simulink model "eurlerAngles_sensor_fusion"  (R2021a)
settings: Solver=FixedStepAuto  StartTime=0.0  StopTime=2000  RelTol=1e-3  EnableMultiTasking=on
undefined symbols (not defined in the file): DiscIntNeverNeededParam
libraries: bbblueCommlib x15, bbblueBasicLib x1, bbblueSensorLib x1
settings Model: ExtModeTrigDuration=100  Creator=Zein  LastModifiedBy=zein
settings SolverCC: AlgebraicLoopSolver=TrustRegion  PositivePriorityOrder=on
settings OptimizationCC: EnhancedBackFolding=on  PassReuseOutputArgsAs=Individual arguments  ZeroExternalMemoryAtStartup=off  ZeroInternalMemoryAtStartup=off  MaxStackSize=64  OptimizeBlockOrder=speed  DifferentSizesBufferReuse=on  OptimizationCustomize=off  EfficientTunableParamExpr=on
settings DebuggingCC: ParameterTunabilityLossMsg=error  SFMachineParentedDataDiag=warning
settings HardwareCC: ProdBitPerPointer=32  ProdBitPerSizeT=32  ProdBitPerPtrDiffT=32  ProdLargestAtomicInteger=Long  ProdLargestAtomicFloat=Double  ProdWordSize=32  ProdHWDeviceType=ARM Compatible->ARM Cortex
settings SFSimCC: MATLABDynamicMemAlloc=off
settings RTWCC: SystemTargetFile=ert.tlc  HardwareBoard=BeagleBone Blue  TLCOptions="-aInlineSetEventsForThisBaseRateFcn=TLC_FALSE -aSuppressMultiTaskScheduler=TLC_FALSE  -aRateBasedStepFcn=0"  TemplateMakefile=ert_default_tmf  Toolchain=GNU GCC BeagleBone Blue
settings CodeAppCC: ForceParamTrailComments=on  IgnoreCustomStorageClasses=off  OperatorAnnotations=on  SimulinkDataObjDesc=on  SFDataObjDesc=on  InsertBlockDesc=on
settings ERTTargetCC: MatFileLogging=on  SupportVariableSizeSignals=on

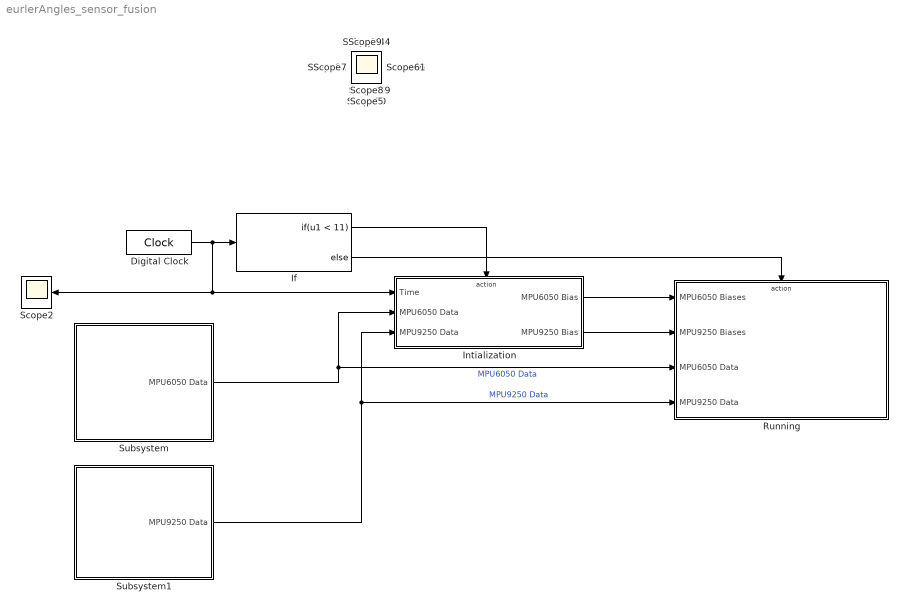
== system eurlerAngles_sensor_fusion ==
  Digital Clock : DigitalClock  SampleTime=0.1
  If : If  IfExpression=u1 < 11
  Intialization : Subsystem  TreatAsAtomicUnit=on
  Running : Subsystem  TreatAsAtomicUnit=on
  Scope{,1..22} (23 alike) : Scope
  Subsystem : Subsystem
  Subsystem1 : Subsystem
  wires:
  If/1 -> Intialization/Action
  Digital Clock/1 -> Scope2/1, Intialization/1(Time), If/1
  If/2 -> Running/Action
  Intialization/1(MPU6050 Bias) -> Running/1(MPU6050 Biases)
  Intialization/2(MPU9250 Bias) -> Running/2(MPU9250 Biases)
  Subsystem/1(MPU6050 Data) -> Intialization/2(MPU6050 Data), Running/3(MPU6050 Data)  "MPU6050 Data"
  Subsystem1/1(MPU9250 Data) -> Intialization/3(MPU9250 Data), Running/4(MPU9250 Data)  "MPU9250 Data"

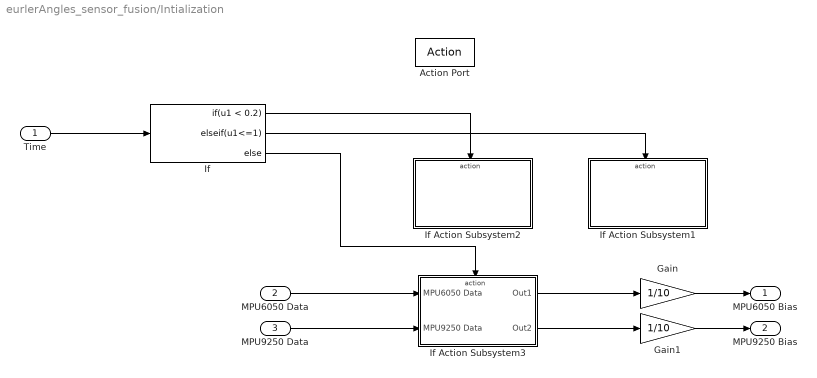
== system eurlerAngles_sensor_fusion/Intialization ==
  Time : Inport
  MPU6050 Data : Inport  Port=2
  MPU9250 Data : Inport  Port=3
  Action Port : ActionPort  ActionPortLabel=if(u1 < 11)
  Gain : Gain  Gain=1/10
  Gain1 : Gain  Gain=1/10
  If : If  IfExpression=u1 < 0.2  ElseIfExpressions=u1<=1
  If Action Subsystem1 : Subsystem  TreatAsAtomicUnit=on
  If Action Subsystem2 : Subsystem  TreatAsAtomicUnit=on
  If Action Subsystem3 : Subsystem  TreatAsAtomicUnit=on
  MPU6050 Bias : Outport
  MPU9250 Bias : Outport  Port=2
  wires:
  Time/1 -> If/1
  If/1 -> If Action Subsystem2/Action
  If/2 -> If Action Subsystem1/Action
  If/3 -> If Action Subsystem3/Action
  If Action Subsystem3/1(Out1) -> Gain/1
  Gain/1 -> MPU6050 Bias/1
  If Action Subsystem3/2(Out2) -> Gain1/1
  Gain1/1 -> MPU9250 Bias/1
  MPU9250 Data/1 -> If Action Subsystem3/2(MPU9250 Data)
  MPU6050 Data/1 -> If Action Subsystem3/1(MPU6050 Data)

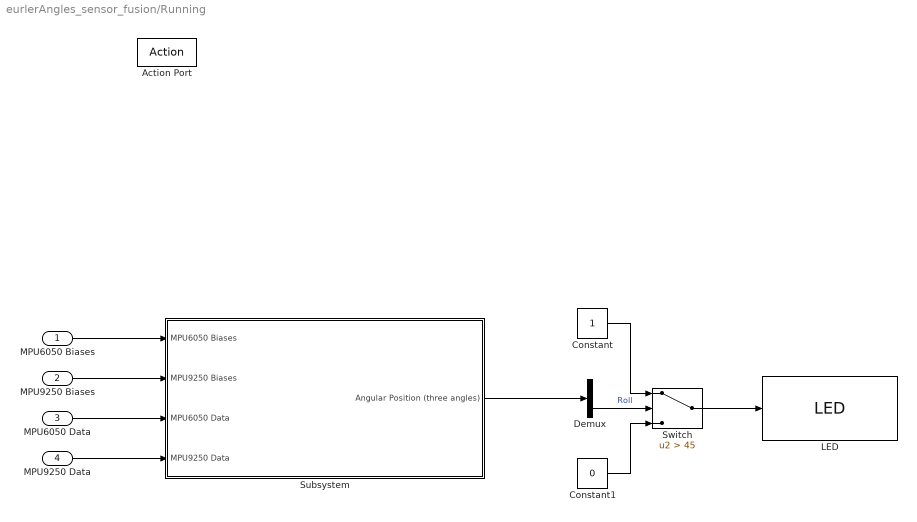
== system eurlerAngles_sensor_fusion/Running ==
  MPU6050 Biases : Inport
  MPU9250 Biases : Inport  Port=2
  MPU6050 Data : Inport  Port=3
  MPU9250 Data : Inport  Port=4
  Action Port : ActionPort  ActionPortLabel=else
  Constant : Constant  OutDataTypeStr=uint8
  Constant1 : Constant  Value=0  OutDataTypeStr=uint8
  Demux : Demux  Outputs=3
  LED : bbblueBasicLib/LED  LED=Red
      settings: SourceProductBaseCode=SC_BEAGLEBONE_BLUE
  Subsystem : Subsystem
  Switch : Switch  Criteria=u2 > Threshold  Threshold=45
  wires:
  Demux/3 -> Switch/2  "Roll"
  Switch/1 -> LED/1
  Constant/1 -> Switch/1
  Constant1/1 -> Switch/3
  MPU6050 Biases/1 -> Subsystem/1(MPU6050 Biases)
  MPU9250 Biases/1 -> Subsystem/2(MPU9250 Biases)
  MPU6050 Data/1 -> Subsystem/3(MPU6050 Data)
  MPU9250 Data/1 -> Subsystem/4(MPU9250 Data)
  Subsystem/1(Angular Position (three angles)) -> Demux/1

== system eurlerAngles_sensor_fusion/Subsystem ==
  MPU6050_Accelerometer : Subsystem
  MPU6050_Gyroscope : Subsystem
  Mux : Mux  Inputs=3
  Mux1 : Mux  Inputs=3
  Mux2 : Mux  Inputs=2
  MPU6050 Data : Outport
  wires:
  Mux/1 -> Mux2/1
  Mux1/1 -> Mux2/2
  Mux2/1 -> MPU6050 Data/1
  MPU6050_Accelerometer/1(Out4) -> Mux/3  "x"
  MPU6050_Accelerometer/2(Out5) -> Mux/1  "y"
  MPU6050_Accelerometer/3(Out6) -> Mux/2  "z"
  MPU6050_Gyroscope/2(Out2) -> Mux1/1  "y"
  MPU6050_Gyroscope/1(Out1) -> Mux1/3  "x"
  MPU6050_Gyroscope/3(Out3) -> Mux1/2  "z"

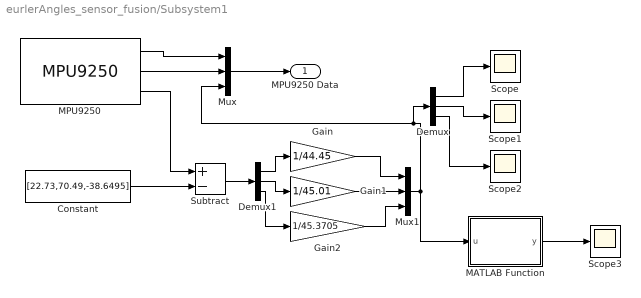
== system eurlerAngles_sensor_fusion/Subsystem1 ==
  Constant : Constant  Value=[22.73,70.49,-38.6495]
  Demux : Demux  Outputs=3
  Demux1 : Demux  Outputs=3
  Gain : Gain  Gain=1/44.45
  Gain1 : Gain  Gain=1/45.01
  Gain2 : Gain  Gain=1/45.3705
  MATLAB Function : MATLAB Function  TreatAsAtomicUnit=on
  MPU9250 : bbblueSensorLib/MPU9250  OperationMode=Random  Accel=on  AngularRate=on  Ak8963Field=on  EulerAngles=on  Quat=off  AccelRange=2G  Acceldlpf=3  GyroRange=250 dps  Gyrodlpf=3  DmpOdr=200 Hz  SampleTime=0.1
      settings: SourceProductBaseCode=SC_BEAGLEBONE_BLUE
  Mux : Mux  Inputs=3
  Mux1 : Mux  Inputs=3
  Scope{,1..3} (4 alike) : Scope
  Subtract : Sum  Inputs=+-
  MPU9250 Data : Outport
  wires:
  MPU9250/1 -> Mux/1
  MPU9250/2 -> Mux/2
  Mux/1 -> MPU9250 Data/1
  Constant/1 -> Subtract/2
  Subtract/1 -> Demux1/1
  MPU9250/3 -> Subtract/1
  Demux/1 -> Scope/1
  Demux/2 -> Scope1/1
  Demux/3 -> Scope2/1
  Demux1/1 -> Gain/1
  Demux1/2 -> Gain1/1
  Demux1/3 -> Gain2/1
  Gain/1 -> Mux1/1
  Gain1/1 -> Mux1/2
  Gain2/1 -> Mux1/3
  Mux1/1 -> MATLAB Function/1(u), Demux/1, Mux/3
  MATLAB Function/1(y) -> Scope3/1

== system eurlerAngles_sensor_fusion/Intialization/If Action Subsystem1 ==
  Action Port : ActionPort  ActionPortLabel=elseif(u1<=1)
  Constant : Constant  Value=0
  Constant1 : Constant  Value=3
  I2C Master Write : bbblueCommlib/I2C Master Write  I2CModule=1  Mode=Master  SlaveAddress=0x69  SlaveByteOrder=BigEndian  Direction=Transmitter  RegisterAddressMode=on  RegisterAddress=107  SlaveDataType=uint8  DataLength=1  NoAck=off  RepeatedStart=off  OutputStatus=off
      settings: SourceProductBaseCode=SC_BEAGLEBONE_BLUE
  I2C Master Write1 : bbblueCommlib/I2C Master Write  I2CModule=1  Mode=Master  SlaveAddress=0x69  SlaveByteOrder=BigEndian  Direction=Transmitter  RegisterAddressMode=on  RegisterAddress=26  SlaveDataType=uint8  DataLength=1  NoAck=off  RepeatedStart=off  OutputStatus=off
      settings: SourceProductBaseCode=SC_BEAGLEBONE_BLUE
  wires:
  Constant/1 -> I2C Master Write/1
  Constant1/1 -> I2C Master Write1/1

== system eurlerAngles_sensor_fusion/Intialization/If Action Subsystem2 ==
  Action Port : ActionPort  ActionPortLabel=if(u1 < 0.2)
  Constant : Constant  Value=80
  I2C Master Write : bbblueCommlib/I2C Master Write  I2CModule=1  Mode=Master  SlaveAddress=0x69  SlaveByteOrder=BigEndian  Direction=Transmitter  RegisterAddressMode=on  RegisterAddress=107  SlaveDataType=uint8  DataLength=1  NoAck=off  RepeatedStart=off  OutputStatus=off
      settings: SourceProductBaseCode=SC_BEAGLEBONE_BLUE
  wires:
  Constant/1 -> I2C Master Write/1

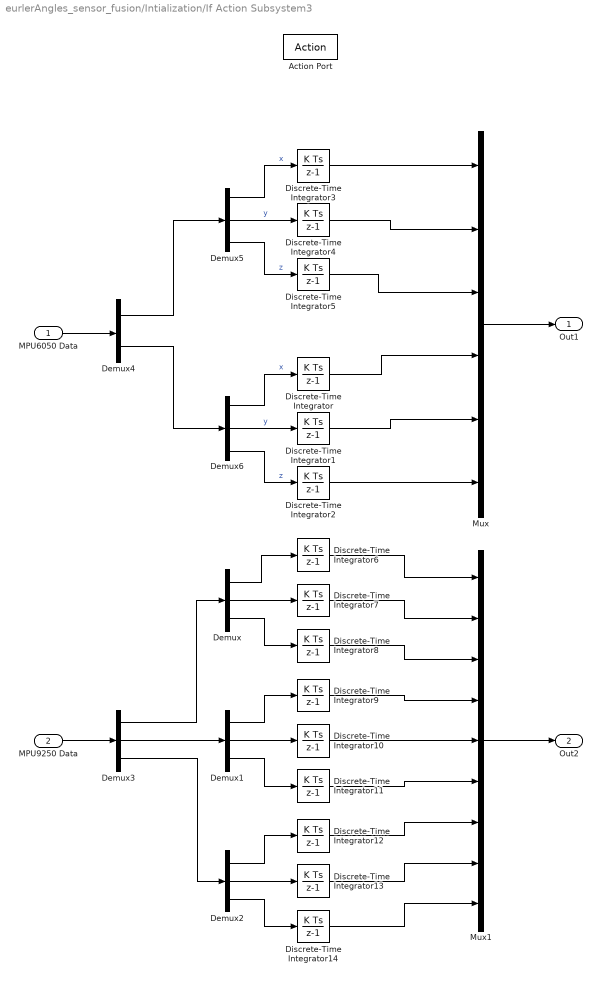
== system eurlerAngles_sensor_fusion/Intialization/If Action Subsystem3 ==
  MPU6050 Data : Inport
  MPU9250 Data : Inport  Port=2
  Action Port : ActionPort  ActionPortLabel=else
  Demux{,1..3,5..6} (6 alike) : Demux  Outputs=3
  Demux4 : Demux  Outputs=2
  Discrete-Time Integrator{,1..14} (15 alike) : DiscreteIntegrator  SampleTime=-1  ICPrevOutput=DiscIntNeverNeededParam  ICPrevScaledInput=DiscIntNeverNeededParam
  Mux : Mux  Inputs=6
  Mux1 : Mux  Inputs=9
  Out1 : Outport
  Out2 : Outport  Port=2
  wires:
  Demux6/1 -> Discrete-Time Integrator/1  "x"
  Demux6/2 -> Discrete-Time Integrator1/1  "y"
  Demux6/3 -> Discrete-Time Integrator2/1  "z"
  Demux5/1 -> Discrete-Time Integrator3/1  "x"
  Demux5/2 -> Discrete-Time Integrator4/1  "y"
  Demux5/3 -> Discrete-Time Integrator5/1  "z"
  Mux/1 -> Out1/1
  Discrete-Time Integrator3/1 -> Mux/1
  Discrete-Time Integrator4/1 -> Mux/2
  Discrete-Time Integrator5/1 -> Mux/3
  Discrete-Time Integrator/1 -> Mux/4
  Discrete-Time Integrator1/1 -> Mux/5
  Discrete-Time Integrator2/1 -> Mux/6
  Demux3/1 -> Demux/1
  Demux3/2 -> Demux1/1
  Demux3/3 -> Demux2/1
  Mux1/1 -> Out2/1
  Demux/1 -> Discrete-Time Integrator6/1
  Demux/2 -> Discrete-Time Integrator7/1
  Demux/3 -> Discrete-Time Integrator8/1
  Demux1/1 -> Discrete-Time Integrator9/1
  Demux1/2 -> Discrete-Time Integrator10/1
  Demux1/3 -> Discrete-Time Integrator11/1
  Demux2/2 -> Discrete-Time Integrator13/1
  Demux2/1 -> Discrete-Time Integrator12/1
  Demux2/3 -> Discrete-Time Integrator14/1
  Discrete-Time Integrator10/1 -> Mux1/5
  Discrete-Time Integrator9/1 -> Mux1/4
  Discrete-Time Integrator8/1 -> Mux1/3
  Discrete-Time Integrator7/1 -> Mux1/2
  Discrete-Time Integrator6/1 -> Mux1/1
  Discrete-Time Integrator11/1 -> Mux1/6
  Discrete-Time Integrator12/1 -> Mux1/7
  Discrete-Time Integrator13/1 -> Mux1/8
  Discrete-Time Integrator14/1 -> Mux1/9
  MPU9250 Data/1 -> Demux3/1
  Demux4/1 -> Demux5/1
  Demux4/2 -> Demux6/1
  MPU6050 Data/1 -> Demux4/1

== system eurlerAngles_sensor_fusion/Running/Subsystem ==
  MPU6050 Biases : Inport
  MPU9250 Biases : Inport  Port=2
  MPU6050 Data : Inport  Port=3
  MPU9250 Data : Inport  Port=4
  Apply accel+gyro+mag composition : Subsystem
  Remove Bias : Subsystem
  Angular Position (three angles) : Outport
  wires:
  Remove Bias/1(MPU6050 Accel) -> Apply accel+gyro+mag composition/1(MPU6050 Accel)
  Remove Bias/3(MPU9250 Accel) -> Apply accel+gyro+mag composition/3(MPU9250 Accel)
  Remove Bias/4(MPU9250 Gyro) -> Apply accel+gyro+mag composition/4(In4)
  Remove Bias/6(MPU6050 Initial Accel) -> Apply accel+gyro+mag composition/6(MPU6050 Initial Accel)
  Remove Bias/7(MPU9250 Initial Accel) -> Apply accel+gyro+mag composition/7(MPU9250 Initial Accel)
  MPU9250 Data/1 -> Remove Bias/4(MPU9250 Data)
  Remove Bias/2(MPU6050 Gyro) -> Apply accel+gyro+mag composition/2(MPU6050 Gyro)
  Remove Bias/8(MPU9250 Initial Mag) -> Apply accel+gyro+mag composition/8(MPU9250 Initial Mag)
  Remove Bias/5(MPU9250 Mag) -> Apply accel+gyro+mag composition/5(" MPU9250 Mag")
  MPU6050 Data/1 -> Remove Bias/3(MPU6050 Data)
  MPU6050 Biases/1 -> Remove Bias/1(MPU6050 Biases)
  MPU9250 Biases/1 -> Remove Bias/2(MPU9250 Biases)
  Apply accel+gyro+mag composition/1(Out1) -> Angular Position (three angles)/1  "Angular Position (three angles)"

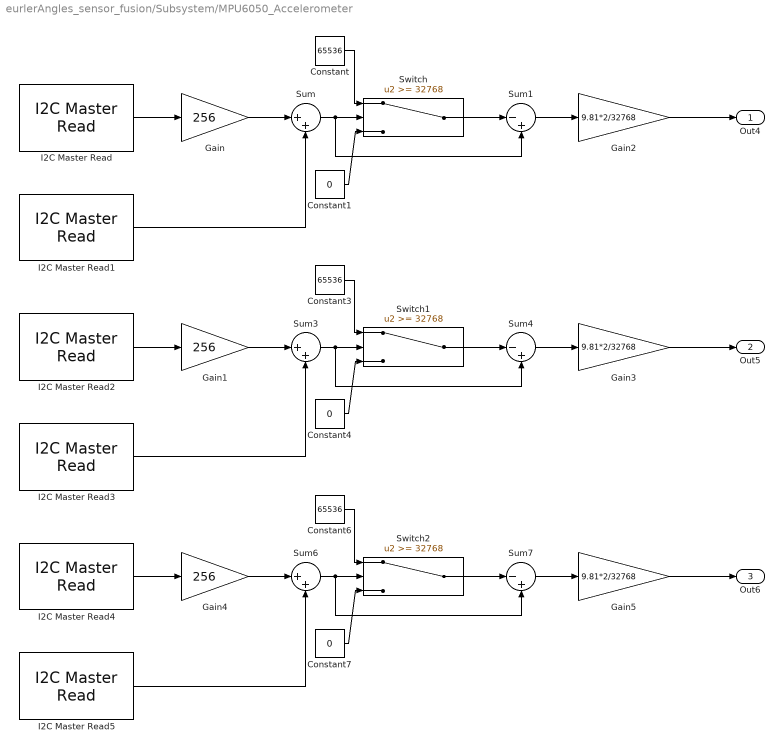
== system eurlerAngles_sensor_fusion/Subsystem/MPU6050_Accelerometer ==
  Constant : Constant  Value=65536
  Constant1 : Constant  Value=0
  Constant3 : Constant  Value=65536
  Constant4 : Constant  Value=0
  Constant6 : Constant  Value=65536
  Constant7 : Constant  Value=0
  Gain : Gain  Gain=256
  Gain1 : Gain  Gain=256
  Gain2 : Gain  Gain=9.81*2/32768
  Gain3 : Gain  Gain=9.81*2/32768
  Gain4 : Gain  Gain=256
  Gain5 : Gain  Gain=9.81*2/32768
  I2C Master Read : bbblueCommlib/I2C Master Read  I2CModule=1  Mode=Master  SlaveAddress=0x69  SlaveByteOrder=BigEndian  Direction=Receiver  RegisterAddressMode=on  RegisterAddress=59  SlaveDataType=int8  DataLength=1  NoAck=off  RepeatedStart=off  OutputStatus=off  SampleTime=0.1
      settings: SourceProductBaseCode=SC_BEAGLEBONE_BLUE
  I2C Master Read1 : bbblueCommlib/I2C Master Read  I2CModule=1  Mode=Master  SlaveAddress=0x69  SlaveByteOrder=BigEndian  Direction=Receiver  RegisterAddressMode=on  RegisterAddress=60  SlaveDataType=int8  DataLength=1  NoAck=off  RepeatedStart=off  OutputStatus=off  SampleTime=0.1
      settings: SourceProductBaseCode=SC_BEAGLEBONE_BLUE
  I2C Master Read2 : bbblueCommlib/I2C Master Read  I2CModule=1  Mode=Master  SlaveAddress=0x69  SlaveByteOrder=BigEndian  Direction=Receiver  RegisterAddressMode=on  RegisterAddress=61  SlaveDataType=int8  DataLength=1  NoAck=off  RepeatedStart=off  OutputStatus=off  SampleTime=0.1
      settings: SourceProductBaseCode=SC_BEAGLEBONE_BLUE
  I2C Master Read3 : bbblueCommlib/I2C Master Read  I2CModule=1  Mode=Master  SlaveAddress=0x69  SlaveByteOrder=BigEndian  Direction=Receiver  RegisterAddressMode=on  RegisterAddress=62  SlaveDataType=int8  DataLength=1  NoAck=off  RepeatedStart=off  OutputStatus=off  SampleTime=0.1
      settings: SourceProductBaseCode=SC_BEAGLEBONE_BLUE
  I2C Master Read4 : bbblueCommlib/I2C Master Read  I2CModule=1  Mode=Master  SlaveAddress=0x69  SlaveByteOrder=BigEndian  Direction=Receiver  RegisterAddressMode=on  RegisterAddress=63  SlaveDataType=int8  DataLength=1  NoAck=off  RepeatedStart=off  OutputStatus=off  SampleTime=0.1
      settings: SourceProductBaseCode=SC_BEAGLEBONE_BLUE
  I2C Master Read5 : bbblueCommlib/I2C Master Read  I2CModule=1  Mode=Master  SlaveAddress=0x69  SlaveByteOrder=BigEndian  Direction=Receiver  RegisterAddressMode=on  RegisterAddress=64  SlaveDataType=int8  DataLength=1  NoAck=off  RepeatedStart=off  OutputStatus=off  SampleTime=0.1
      settings: SourceProductBaseCode=SC_BEAGLEBONE_BLUE
  Sum : Sum  Inputs=|++
  Sum1 : Sum  Inputs=|-+
  Sum3 : Sum  Inputs=|++
  Sum4 : Sum  Inputs=|-+
  Sum6 : Sum  Inputs=|++
  Sum7 : Sum  Inputs=|-+
  Switch : Switch  Threshold=32768
  Switch1 : Switch  Threshold=32768
  Switch2 : Switch  Threshold=32768
  Out4 : Outport
  Out5 : Outport  Port=2
  Out6 : Outport  Port=3
  wires:
  Constant/1 -> Switch/1
  I2C Master Read1/1 -> Sum/2
  I2C Master Read2/1 -> Gain1/1
  Sum/1 -> Switch/2, Sum1/2
  Sum4/1 -> Gain3/1
  Constant3/1 -> Switch1/1
  Sum6/1 -> Switch2/2, Sum7/2
  I2C Master Read4/1 -> Gain4/1
  Gain1/1 -> Sum3/1
  Switch/1 -> Sum1/1
  I2C Master Read5/1 -> Sum6/2
  Constant6/1 -> Switch2/1
  Switch2/1 -> Sum7/1
  Gain4/1 -> Sum6/1
  Switch1/1 -> Sum4/1
  I2C Master Read3/1 -> Sum3/2
  Gain2/1 -> Out4/1
  Constant1/1 -> Switch/3
  Constant4/1 -> Switch1/3
  Sum1/1 -> Gain2/1
  Sum7/1 -> Gain5/1
  Gain5/1 -> Out6/1
  I2C Master Read/1 -> Gain/1
  Gain/1 -> Sum/1
  Sum3/1 -> Sum4/2, Switch1/2
  Gain3/1 -> Out5/1
  Constant7/1 -> Switch2/3

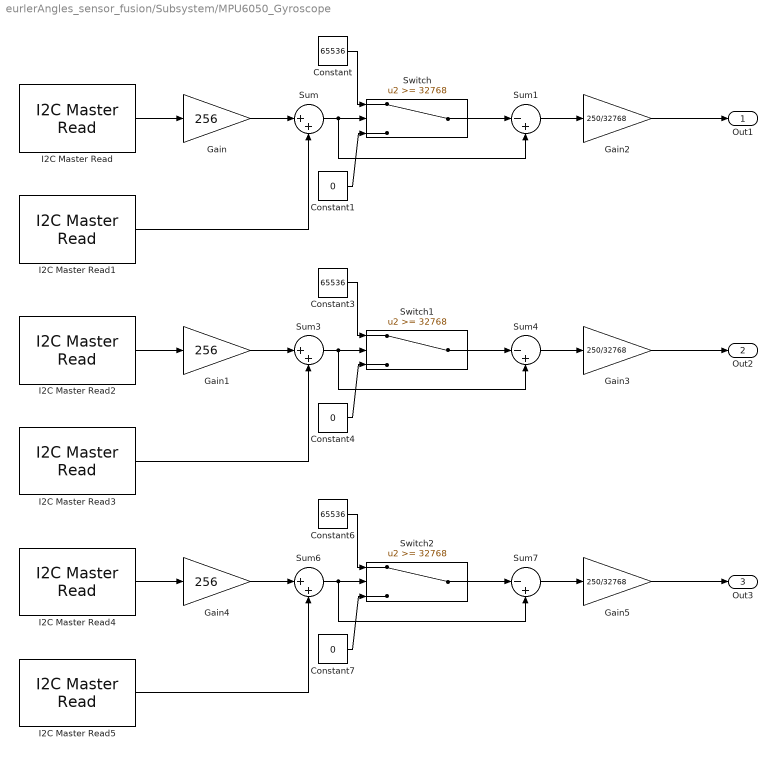
== system eurlerAngles_sensor_fusion/Subsystem/MPU6050_Gyroscope ==
  Constant : Constant  Value=65536
  Constant1 : Constant  Value=0
  Constant3 : Constant  Value=65536
  Constant4 : Constant  Value=0
  Constant6 : Constant  Value=65536
  Constant7 : Constant  Value=0
  Gain : Gain  Gain=256
  Gain1 : Gain  Gain=256
  Gain2 : Gain  Gain=250/32768
  Gain3 : Gain  Gain=250/32768
  Gain4 : Gain  Gain=256
  Gain5 : Gain  Gain=250/32768
  I2C Master Read : bbblueCommlib/I2C Master Read  I2CModule=1  Mode=Master  SlaveAddress=0x69  SlaveByteOrder=BigEndian  Direction=Receiver  RegisterAddressMode=on  RegisterAddress=67  SlaveDataType=int8  DataLength=1  NoAck=off  RepeatedStart=off  OutputStatus=off  SampleTime=0.1
      settings: SourceProductBaseCode=SC_BEAGLEBONE_BLUE
  I2C Master Read1 : bbblueCommlib/I2C Master Read  I2CModule=1  Mode=Master  SlaveAddress=0x69  SlaveByteOrder=BigEndian  Direction=Receiver  RegisterAddressMode=on  RegisterAddress=68  SlaveDataType=int8  DataLength=1  NoAck=off  RepeatedStart=off  OutputStatus=off  SampleTime=0.1
      settings: SourceProductBaseCode=SC_BEAGLEBONE_BLUE
  I2C Master Read2 : bbblueCommlib/I2C Master Read  I2CModule=1  Mode=Master  SlaveAddress=0x69  SlaveByteOrder=BigEndian  Direction=Receiver  RegisterAddressMode=on  RegisterAddress=69  SlaveDataType=int8  DataLength=1  NoAck=off  RepeatedStart=off  OutputStatus=off  SampleTime=0.1
      settings: SourceProductBaseCode=SC_BEAGLEBONE_BLUE
  I2C Master Read3 : bbblueCommlib/I2C Master Read  I2CModule=1  Mode=Master  SlaveAddress=0x69  SlaveByteOrder=BigEndian  Direction=Receiver  RegisterAddressMode=on  RegisterAddress=70  SlaveDataType=int8  DataLength=1  NoAck=off  RepeatedStart=off  OutputStatus=off  SampleTime=0.1
      settings: SourceProductBaseCode=SC_BEAGLEBONE_BLUE
  I2C Master Read4 : bbblueCommlib/I2C Master Read  I2CModule=1  Mode=Master  SlaveAddress=0x69  SlaveByteOrder=BigEndian  Direction=Receiver  RegisterAddressMode=on  RegisterAddress=71  SlaveDataType=int8  DataLength=1  NoAck=off  RepeatedStart=off  OutputStatus=off  SampleTime=0.1
      settings: SourceProductBaseCode=SC_BEAGLEBONE_BLUE
  I2C Master Read5 : bbblueCommlib/I2C Master Read  I2CModule=1  Mode=Master  SlaveAddress=0x69  SlaveByteOrder=BigEndian  Direction=Receiver  RegisterAddressMode=on  RegisterAddress=72  SlaveDataType=int8  DataLength=1  NoAck=off  RepeatedStart=off  OutputStatus=off  SampleTime=0.1
      settings: SourceProductBaseCode=SC_BEAGLEBONE_BLUE
  Sum : Sum  Inputs=|++
  Sum1 : Sum  Inputs=|-+
  Sum3 : Sum  Inputs=|++
  Sum4 : Sum  Inputs=|-+
  Sum6 : Sum  Inputs=|++
  Sum7 : Sum  Inputs=|-+
  Switch : Switch  Threshold=32768
  Switch1 : Switch  Threshold=32768
  Switch2 : Switch  Threshold=32768
  Out1 : Outport
  Out2 : Outport  Port=2
  Out3 : Outport  Port=3
  wires:
  I2C Master Read3/1 -> Sum3/2
  Sum4/1 -> Gain3/1
  Sum/1 -> Switch/2, Sum1/2
  I2C Master Read/1 -> Gain/1
  Sum3/1 -> Sum4/2, Switch1/2
  I2C Master Read1/1 -> Sum/2
  Constant/1 -> Switch/1
  Gain/1 -> Sum/1
  Sum6/1 -> Switch2/2, Sum7/2
  Constant1/1 -> Switch/3
  Switch/1 -> Sum1/1
  Sum1/1 -> Gain2/1
  I2C Master Read4/1 -> Gain4/1
  Switch2/1 -> Sum7/1
  I2C Master Read2/1 -> Gain1/1
  Switch1/1 -> Sum4/1
  Constant4/1 -> Switch1/3
  Gain1/1 -> Sum3/1
  Constant3/1 -> Switch1/1
  Gain4/1 -> Sum6/1
  Sum7/1 -> Gain5/1
  Gain2/1 -> Out1/1
  Constant6/1 -> Switch2/1
  I2C Master Read5/1 -> Sum6/2
  Constant7/1 -> Switch2/3
  Gain3/1 -> Out2/1
  Gain5/1 -> Out3/1

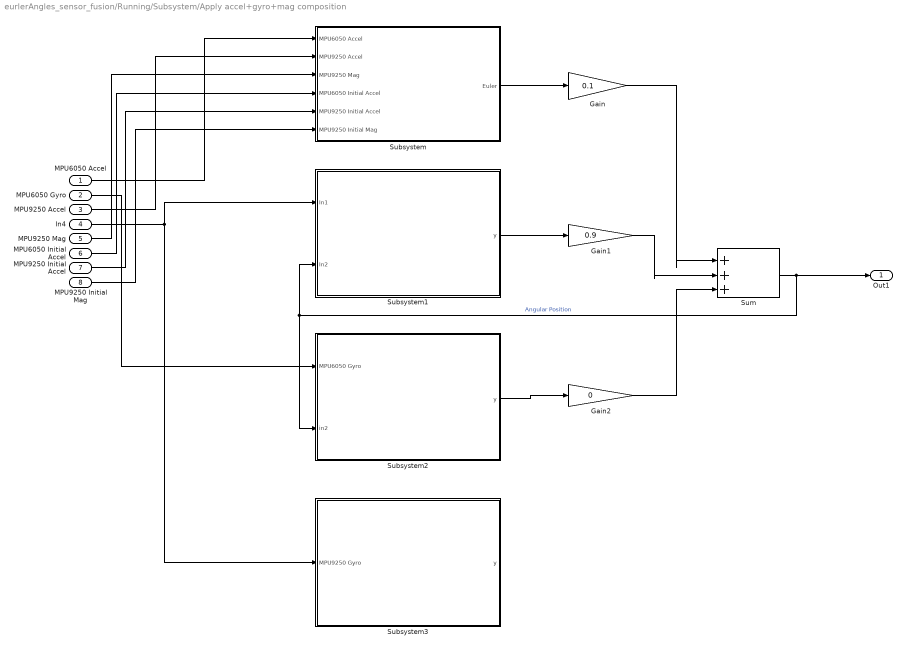
== system eurlerAngles_sensor_fusion/Running/Subsystem/Apply accel+gyro+mag composition ==
  MPU6050 Accel : Inport
  MPU6050 Gyro : Inport  Port=2
  MPU9250 Accel : Inport  Port=3
  In4 : Inport  Port=4
  " MPU9250 Mag" : Inport  Port=5
  MPU6050 Initial Accel : Inport  Port=6
  MPU9250 Initial Accel : Inport  Port=7
  MPU9250 Initial Mag : Inport  Port=8
  Gain : Gain  Gain=0.1
  Gain1 : Gain  Gain=0.9
  Gain2 : Gain  Gain=0
  Subsystem : Subsystem
  Subsystem1 : Subsystem
  Subsystem2 : Subsystem
  Subsystem3 : Subsystem
  Sum : Sum  Inputs=|+++
  Out1 : Outport
  wires:
  Gain2/1 -> Sum/3
  Subsystem/1(Euler) -> Gain/1
  Gain1/1 -> Sum/2
  Sum/1 -> Subsystem2/2(in2), Subsystem1/2(In2), Out1/1  "Angular Position"
  In4/1 -> Subsystem3/1(MPU9250 Gyro), Subsystem1/1(In1)
  Gain/1 -> Sum/1
  MPU6050 Gyro/1 -> Subsystem2/1(MPU6050 Gyro)
  Subsystem1/1(y) -> Gain1/1
  Subsystem2/1(y) -> Gain2/1
  MPU9250 Initial Accel/1 -> Subsystem/5(MPU9250 Initial Accel)
  MPU6050 Accel/1 -> Subsystem/1(MPU6050 Accel)
  MPU6050 Initial Accel/1 -> Subsystem/4(MPU6050 Initial Accel)
  MPU9250 Accel/1 -> Subsystem/2(MPU9250 Accel)
  " MPU9250 Mag"/1 -> Subsystem/3(" MPU9250 Mag")
  MPU9250 Initial Mag/1 -> Subsystem/6(MPU9250 Initial Mag)

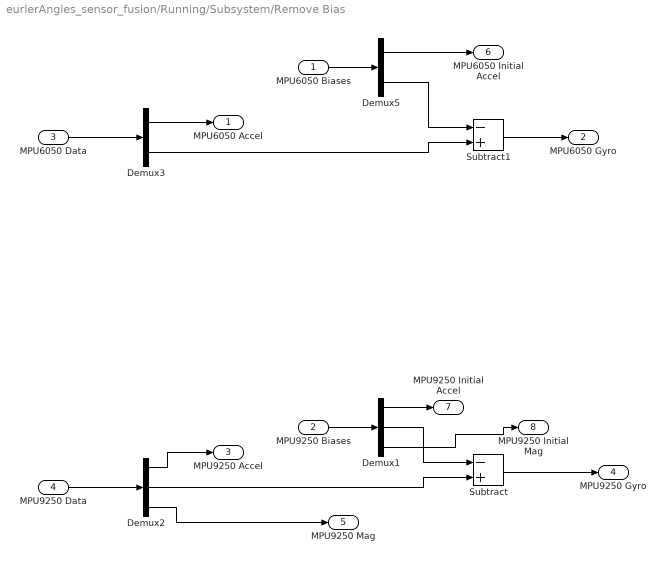
== system eurlerAngles_sensor_fusion/Running/Subsystem/Remove Bias ==
  MPU6050 Biases : Inport
  MPU9250 Biases : Inport  Port=2
  MPU6050 Data : Inport  Port=3
  MPU9250 Data : Inport  Port=4
  Demux1 : Demux  Outputs=3
  Demux2 : Demux  Outputs=3
  Demux3 : Demux  Outputs=2
  Demux5 : Demux  Outputs=2
  Subtract : Sum  Inputs=-+
  Subtract1 : Sum  Inputs=-+
  MPU6050 Accel : Outport
  MPU6050 Gyro : Outport  Port=2
  MPU9250 Accel : Outport  Port=3
  MPU9250 Gyro : Outport  Port=4
  MPU9250 Mag : Outport  Port=5
  MPU6050 Initial Accel : Outport  Port=6
  MPU9250 Initial Accel : Outport  Port=7
  MPU9250 Initial Mag : Outport  Port=8
  wires:
  Demux5/2 -> Subtract1/1
  MPU9250 Data/1 -> Demux2/1
  Demux2/1 -> MPU9250 Accel/1
  MPU6050 Biases/1 -> Demux5/1
  Demux2/3 -> MPU9250 Mag/1
  Subtract1/1 -> MPU6050 Gyro/1
  MPU6050 Data/1 -> Demux3/1
  Demux3/2 -> Subtract1/2
  MPU9250 Biases/1 -> Demux1/1
  Demux3/1 -> MPU6050 Accel/1
  Demux1/2 -> Subtract/1
  Demux2/2 -> Subtract/2
  Subtract/1 -> MPU9250 Gyro/1
  Demux5/1 -> MPU6050 Initial Accel/1
  Demux1/1 -> MPU9250 Initial Accel/1
  Demux1/3 -> MPU9250 Initial Mag/1

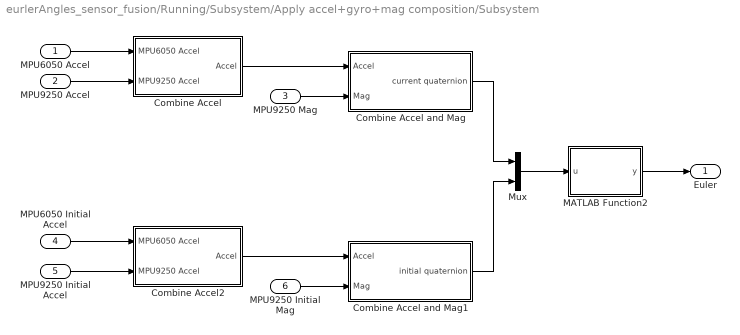
== system eurlerAngles_sensor_fusion/Running/Subsystem/Apply accel+gyro+mag composition/Subsystem ==
  MPU6050 Accel : Inport
  MPU9250 Accel : Inport  Port=2
  " MPU9250 Mag" : Inport  Port=3
  MPU6050 Initial Accel : Inport  Port=4
  MPU9250 Initial Accel : Inport  Port=5
  MPU9250 Initial Mag : Inport  Port=6
  Combine Accel : Subsystem
  Combine Accel and Mag : Subsystem
  Combine Accel and Mag1 : Subsystem
  Combine Accel2 : Subsystem
  MATLAB Function2 : MATLAB Function  TreatAsAtomicUnit=on
  Mux : Mux  Inputs=2
  Euler : Outport
  wires:
  " MPU9250 Mag"/1 -> Combine Accel and Mag/2(" Mag")
  Combine Accel/1(Accel) -> Combine Accel and Mag/1(Accel)
  Combine Accel and Mag1/1(initial quaternion) -> Mux/2
  MPU6050 Initial Accel/1 -> Combine Accel2/1(MPU6050 Accel)
  Mux/1 -> MATLAB Function2/1(u)
  MPU9250 Accel/1 -> Combine Accel/2(MPU9250 Accel)
  Combine Accel2/1(Accel) -> Combine Accel and Mag1/1(Accel)
  Combine Accel and Mag/1(current quaternion) -> Mux/1
  MPU6050 Accel/1 -> Combine Accel/1(MPU6050 Accel)
  MPU9250 Initial Accel/1 -> Combine Accel2/2(MPU9250 Accel)
  MPU9250 Initial Mag/1 -> Combine Accel and Mag1/2(" Mag")
  MATLAB Function2/1(y) -> Euler/1

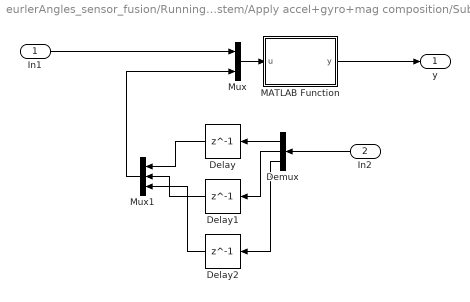
== system eurlerAngles_sensor_fusion/Running/Subsystem/Apply accel+gyro+mag composition/Subsystem1 ==
  In1 : Inport
  In2 : Inport  Port=2
  Delay : Delay  DelayLength=1
  Delay1 : Delay  DelayLength=1
  Delay2 : Delay  DelayLength=1
  Demux : Demux  Outputs=3
  MATLAB Function : MATLAB Function  TreatAsAtomicUnit=on
  Mux : Mux  Inputs=2
  Mux1 : Mux  Inputs=3
  y : Outport
  wires:
  Delay/1 -> Mux1/1
  In1/1 -> Mux/1
  Mux1/1 -> Mux/2
  Mux/1 -> MATLAB Function/1(u)
  Demux/2 -> Delay1/1
  Delay1/1 -> Mux1/2
  Demux/1 -> Delay/1
  Delay2/1 -> Mux1/3
  Demux/3 -> Delay2/1
  MATLAB Function/1(y) -> y/1
  In2/1 -> Demux/1

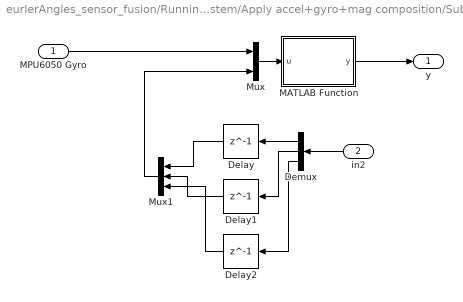
== system eurlerAngles_sensor_fusion/Running/Subsystem/Apply accel+gyro+mag composition/Subsystem2 ==
  MPU6050 Gyro : Inport
  in2 : Inport  Port=2
  Delay : Delay  DelayLength=1
  Delay1 : Delay  DelayLength=1
  Delay2 : Delay  DelayLength=1
  Demux : Demux  Outputs=3
  MATLAB Function : MATLAB Function  TreatAsAtomicUnit=on
  Mux : Mux  Inputs=2
  Mux1 : Mux  Inputs=3
  y : Outport
  wires:
  MATLAB Function/1(y) -> y/1
  Demux/3 -> Delay2/1
  Delay2/1 -> Mux1/3
  Demux/1 -> Delay/1
  Delay1/1 -> Mux1/2
  Demux/2 -> Delay1/1
  Mux/1 -> MATLAB Function/1(u)
  Mux1/1 -> Mux/2
  MPU6050 Gyro/1 -> Mux/1
  Delay/1 -> Mux1/1
  in2/1 -> Demux/1

== system eurlerAngles_sensor_fusion/Running/Subsystem/Apply accel+gyro+mag composition/Subsystem3 ==
  MPU9250 Gyro : Inport
  Delay : Delay  DelayLength=1
  Delay1 : Delay  DelayLength=1
  Delay2 : Delay  DelayLength=1
  Demux : Demux  Outputs=3
  MATLAB Function : MATLAB Function  TreatAsAtomicUnit=on
  Mux : Mux  Inputs=2
  Mux1 : Mux  Inputs=3
  y : Outport
  wires:
  MATLAB Function/1(y) -> Demux/1, y/1
  Demux/3 -> Delay2/1
  Delay2/1 -> Mux1/3
  Demux/1 -> Delay/1
  Delay1/1 -> Mux1/2
  Demux/2 -> Delay1/1
  Mux/1 -> MATLAB Function/1(u)
  Mux1/1 -> Mux/2
  MPU9250 Gyro/1 -> Mux/1
  Delay/1 -> Mux1/1

== system eurlerAngles_sensor_fusion/Running/Subsystem/Apply accel+gyro+mag composition/Subsystem/Combine Accel ==
  MPU6050 Accel : Inport
  MPU9250 Accel : Inport  Port=2
  Add : Sum
  Gain : Gain  Gain=1/2
  Accel : Outport
  wires:
  MPU9250 Accel/1 -> Add/2
  Add/1 -> Gain/1
  Gain/1 -> Accel/1
  MPU6050 Accel/1 -> Add/1

== system eurlerAngles_sensor_fusion/Running/Subsystem/Apply accel+gyro+mag composition/Subsystem/Combine Accel and Mag ==
  Accel : Inport
  " Mag" : Inport  Port=2
  MATLAB Function : MATLAB Function  TreatAsAtomicUnit=on
  MATLAB Function1 : MATLAB Function  TreatAsAtomicUnit=on
  MATLAB Function2 : MATLAB Function  TreatAsAtomicUnit=on
  Mux : Mux  Inputs=2
  current quaternion : Outport
  wires:
  Accel/1 -> MATLAB Function/1(u)
  " Mag"/1 -> MATLAB Function1/1(u)
  Mux/1 -> MATLAB Function2/1(u)
  MATLAB Function2/1(y) -> current quaternion/1
  MATLAB Function/1(y) -> Mux/1
  MATLAB Function1/1(y) -> Mux/2

== system eurlerAngles_sensor_fusion/Running/Subsystem/Apply accel+gyro+mag composition/Subsystem/Combine Accel and Mag1 ==
  Accel : Inport
  " Mag" : Inport  Port=2
  MATLAB Function : MATLAB Function  TreatAsAtomicUnit=on
  MATLAB Function1 : MATLAB Function  TreatAsAtomicUnit=on
  MATLAB Function2 : MATLAB Function  TreatAsAtomicUnit=on
  Mux : Mux  Inputs=2
  initial quaternion : Outport
  wires:
  MATLAB Function1/1(y) -> Mux/2
  MATLAB Function/1(y) -> Mux/1
  MATLAB Function2/1(y) -> initial quaternion/1
  Mux/1 -> MATLAB Function2/1(u)
  " Mag"/1 -> MATLAB Function1/1(u)
  Accel/1 -> MATLAB Function/1(u)

== system eurlerAngles_sensor_fusion/Running/Subsystem/Apply accel+gyro+mag composition/Subsystem/Combine Accel2 ==
  MPU6050 Accel : Inport
  MPU9250 Accel : Inport  Port=2
  Add : Sum
  Gain : Gain  Gain=1/2
  Accel : Outport
  wires:
  Gain/1 -> Accel/1
  Add/1 -> Gain/1
  MPU9250 Accel/1 -> Add/2
  MPU6050 Accel/1 -> Add/1

== matlab function eurlerAngles_sensor_fusion/Running/Subsystem/Apply accel+gyro+mag composition/Subsystem/Combine Accel and Mag/MATLAB Function ==
  data: u input; y output
function y = fcn(u)

y=u/norm(u);

== matlab function eurlerAngles_sensor_fusion/Running/Subsystem/Apply accel+gyro+mag composition/Subsystem/Combine Accel and Mag/MATLAB Function2 ==
  data: u input; y output
function y = fcn(u)

accel=[u(1);u(2);u(3)];
mag=[u(5);u(4);-u(6)];
q = ecompass(accel',mag');
y=compact(q);


% 
% theta=asin(-R(3,1));
% psi=atan2(R(2,1),R(1,1));
% phi=atan2(R(3,2),R(3,3));
% euler=[phi;theta;psi];


% r = ecompass(accel',mag','rotmat')';
% theta = -asin(r(1,3));
% psi = atan2(r(2,3)/cos(theta),r(3,3)/cos(theta));
% rho = atan2(r(1,2)/cos(theta),r(1,1)/cos(theta));
% euler = rad2deg([rho,theta,psi]);

== matlab function eurlerAngles_sensor_fusion/Running/Subsystem/Apply accel+gyro+mag composition/Subsystem1/MATLAB Function ==
  data: u input; y output
function y = fcn(u)

if(length(u)==6) 
    Gyro=[u(1);u(2);u(3)];
    Previous=[u(4);u(5);u(6)];

    ph=Previous(1);
    tet=Previous(2);

    R1=[1,sind(ph)*tand(tet),cosd(ph)*tand(tet);
        0,cosd(ph),-sind(ph);
        0,sind(ph)/cosd(tet),cosd(ph)/cosd(tet)];

    dt=0.1;

    New=Previous+R1*Gyro*dt;
else
    New=[0;0;0];
end

y = New;

== matlab function eurlerAngles_sensor_fusion/Running/Subsystem/Apply accel+gyro+mag composition/Subsystem2/MATLAB Function ==
  data: u input; y output
function y = fcn(u)

if(length(u)==6) 
    Gyro=[u(1);u(2);u(3)];
    Previous=[u(4);u(5);u(6)];

    ph=Previous(1);
    tet=Previous(2);

    R1=[1,sind(ph)*tand(tet),cosd(ph)*tand(tet);
        0,cosd(ph),-sind(ph);
        0,sind(ph)/cosd(tet),cosd(ph)/cosd(tet)];

    dt=0.1;

    New=Previous+R1*Gyro*dt;
else
    New=[0;0;0];
end

y = New;

== matlab function eurlerAngles_sensor_fusion/Running/Subsystem/Apply accel+gyro+mag composition/Subsystem3/MATLAB Function ==
  data: u input; y output
function y = fcn(u)

if(length(u)==6) 
    Gyro=[u(1);u(2);u(3)];
    Previous=[u(4);u(5);u(6)];

    ph=Previous(1);
    tet=Previous(2);

    R1=[1,sind(ph)*tand(tet),cosd(ph)*tand(tet);
        0,cosd(ph),-sind(ph);
        0,sind(ph)/cosd(tet),cosd(ph)/cosd(tet)];

    dt=0.1;

    New=Previous+R1*Gyro*dt;
else
    New=[0;0;0];
end

y = New;

== matlab function eurlerAngles_sensor_fusion/Running/Subsystem/Apply accel+gyro+mag composition/Subsystem/Combine Accel and Mag1/MATLAB Function ==
  data: u input; y output
function y = fcn(u)

y=u/norm(u);

== matlab function eurlerAngles_sensor_fusion/Running/Subsystem/Apply accel+gyro+mag composition/Subsystem/Combine Accel and Mag1/MATLAB Function1 ==
  data: u input; y output
function y = fcn(u)

y=u/norm(u);

== matlab function eurlerAngles_sensor_fusion/Running/Subsystem/Apply accel+gyro+mag composition/Subsystem/Combine Accel and Mag1/MATLAB Function2 ==
  data: u input; y output
function y = fcn(u)

accel=[u(1);u(2);u(3)];
mag=[u(5);u(4);-u(6)];
q = ecompass(accel',mag');

y=compact(q);

== matlab function eurlerAngles_sensor_fusion/Running/Subsystem/Apply accel+gyro+mag composition/Subsystem/Combine Accel and Mag/MATLAB Function1 ==
  data: u input; y output
function y = fcn(u)

y=u/norm(u);

== matlab function eurlerAngles_sensor_fusion/Running/Subsystem/Apply accel+gyro+mag composition/Subsystem/MATLAB Function2 ==
  data: u input; y output
function y = fcn(u)

q2=[u(1),u(2),u(3),u(4)];
q1=[u(5),u(6),u(7),u(8)];

Q1=quaternion(q1);
Q2=quaternion(q2);

R1 = rotmat(Q1,'frame');
R2 = rotmat(Q2,'frame');

R=R1*R2';

theta=asin(-R(3,1));
psi=atan2(R(2,1)/cos(theta),R(1,1)/cos(theta));
phi=atan2(R(3,2)/cos(theta),R(3,3)/cos(theta));
euler=[phi;theta;psi]*180/pi;

y=euler;


% 
% theta=asin(-R(3,1));
% psi=atan2(R(2,1),R(1,1));
% phi=atan2(R(3,2),R(3,3));
% euler=[phi;theta;psi];


% r = ecompass(accel',mag','rotmat')';
% theta = -asin(r(1,3));
% psi = atan2(r(2,3)/cos(theta),r(3,3)/cos(theta));
% rho = atan2(r(1,2)/cos(theta),r(1,1)/cos(theta));
% euler = rad2deg([rho,theta,psi]);

== matlab function eurlerAngles_sensor_fusion/Subsystem1/MATLAB Function ==
  data: u input; y output
function y = fcn(u)

y = norm(u);
